simulink model "echo_effect"  (R2017b)
settings: Solver=VariableStepAuto  StartTime=0.0  StopTime=10.0  RelTol=1e-3
libraries: dspvision x1, dspsnks4 x1
settings Model: Creator=Ross_admin  LastModifiedBy=bugsbunny
settings OptimizationCC: BlockReduction=off  ConditionallyExecuteInputs=off  DefaultParameterBehavior=Inlined
settings DebuggingCC: AlgebraicLoopMsg=none
settings HardwareCC: ProdBitPerPointer=32  ProdBitPerSizeT=32  ProdBitPerPtrDiffT=32  ProdLargestAtomicFloat=None  ProdIntDivRoundTo=Undefined  ProdEndianess=Unspecified  ProdWordSize=32  ProdHWDeviceType=ASIC/FPGA->ASIC/FPGA  TargetBitPerLong=64  TargetBitPerPointer=64  TargetBitPerSizeT=64  TargetBitPerPtrDiffT=64  TargetLongLongMode=on  TargetIntDivRoundTo=Zero  TargetEndianess=LittleEndian  TargetWordSize=64  TargetHWDeviceType=Custom Processor->MATLAB Host Computer  ProdEqTarget=off
settings CodeAppCC: StateflowObjectComments=on

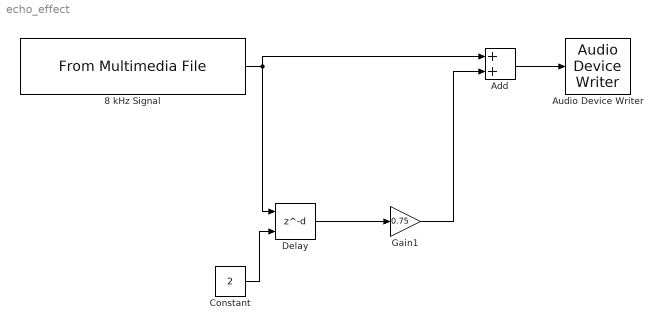
== system echo_effect ==
  8 kHz Signal : dspvision/From Multimedia File  inputFilename=speech_dft_8kHz.wav  loop=on  numPlays=1  outputStreams=Audio only  videoDataType=single  audioDataType=double  inheritSampleTime=on  userDefinedSampleTime=1/30  noAudioOutput=off  isIntensityVideo=off  fourcc=RGB  colorVideoFormat=Separate color signals  outputEOF=off  dataOrg=Column-major  audioFrameSize=1024  computeAudioFrameSize=off  outSamplingMode=Sample based
      settings: SourceProductBaseCode=VP
  Add : Sum
  Audio Device Writer : dspsnks4/Audio Device Writer  Driver=ALSA  Device=Default  InheritSampleRate=on  SampleRate=44100  BitDepth=16-bit integer  BufferSize=4096  NumBuffers=10  DefaultOutputChannelMapping=on  OutputChannelMapping=1:2  OutputNumUnderrunSamples=off  DriverIdx=8  DeviceWarnFlag=''
  Constant : Constant  Value=2
  Delay : Delay  DelayLengthSource=Input port  DelayLength=1  InitialCondition=0
      settings: InputPortMap=u0,p1
  Gain1 : Gain  Gain=0.75
  wires:
  8 kHz Signal/1 -> Add/1, Delay/1
  Constant/1 -> Delay/2
  Add/1 -> Audio Device Writer/1
  Delay/1 -> Gain1/1
  Gain1/1 -> Add/2
